simulink model "TestbedModel_v6"  (R2016a)
settings: Solver=ode23tb  StartTime=0.0  StopTime=20  RelTol=1e-3
undefined symbols (not defined in the file): K, Ki, Kp, magnitude, rev_comms_sink, tau
libraries: DAEMOT_Lib x4
(part 3 of 4)

== system TestbedModel_v6/Data Manager23 ==
  Bus Creator : BusCreator  Inputs=1
  Bus Selector1 : BusSelector  OutputSignals=Voltage [V]
  SubSystem1 : Subsystem
  Data : Outport
  wires:
  SubSystem1/1(Bus) -> Bus Creator/1  "Bus/Voltage [V]"
  Bus Selector1/1 -> SubSystem1/1(Rename)  "<Voltage [V]>"
  [gdata_BusData_Sink] -> Bus Selector1/1  "Bus/Voltage [V]"
  Bus Creator/1 -> Data/1

== system TestbedModel_v6/Data Manager24 ==
  Bus Creator : BusCreator  Inputs=1
  Bus Selector1 : BusSelector  OutputSignals=Speed [rad_s]
  SubSystem1 : Subsystem
  Data : Outport
  wires:
  Bus Creator/1 -> Data/1
  [gdata_ShaftData_Sink] -> Bus Selector1/1  "Shaft/Speed [rad_s]"
  Bus Selector1/1 -> SubSystem1/1(Rename)  "<Speed [rad_s]>"
  SubSystem1/1(Bus) -> Bus Creator/1  "Shaft/Speed [rad_s]"

== system TestbedModel_v6/Data Manager25 ==
  Bus Creator : BusCreator  Inputs=1
  Bus Selector1 : BusSelector  OutputSignals=Speed [rad_s]
  SubSystem1 : Subsystem
  Data : Outport
  wires:
  Bus Creator/1 -> Data/1
  [gdata_ShaftData_Sink] -> Bus Selector1/1  "Shaft/Speed [rad_s]"
  Bus Selector1/1 -> SubSystem1/1(Rename)  "<Speed [rad_s]>"
  SubSystem1/1(Bus) -> Bus Creator/1  "Shaft/Speed [rad_s]"

== system TestbedModel_v6/Data Manager3 ==
  Bus Creator : BusCreator  Inputs=1
  Bus Selector1 : BusSelector  OutputSignals=Voltage Out [V]
  SubSystem1 : Subsystem
  Data : Outport
  wires:
  Bus Creator/1 -> Data/1
  [gdata_ConverterData_Sink] -> Bus Selector1/1  "Converter/Voltage Out [V]"
  Bus Selector1/1 -> SubSystem1/1(Rename)  "<Voltage Out [V]>"
  SubSystem1/1(Bus) -> Bus Creator/1  "Converter/Voltage Out [V]"

== system TestbedModel_v6/Data Manager4 ==
  Bus Creator : BusCreator  Inputs=1
  Bus Selector1 : BusSelector  OutputSignals=Torque [Nm]
  SubSystem1 : Subsystem
  Data : Outport
  wires:
  Bus Creator/1 -> Data/1
  [gdata_MotorData_Sink] -> Bus Selector1/1  "Motor/Torque [Nm]"
  Bus Selector1/1 -> SubSystem1/1(Rename)  "<Torque [Nm]>"
  SubSystem1/1(Bus) -> Bus Creator/1  "Motor/Torque [Nm]"

== system TestbedModel_v6/Data Manager5 ==
  Bus Creator : BusCreator  Inputs=1
  Bus Selector1 : BusSelector  OutputSignals=Torque [Nm]
  SubSystem1 : Subsystem
  Data : Outport
  wires:
  Bus Creator/1 -> Data/1
  [gdata_MotorData_Sink] -> Bus Selector1/1  "Motor/Torque [Nm]"
  Bus Selector1/1 -> SubSystem1/1(Rename)  "<Torque [Nm]>"
  SubSystem1/1(Bus) -> Bus Creator/1  "Motor/Torque [Nm]"

== system TestbedModel_v6/Data Manager6 ==
  Bus Creator : BusCreator  Inputs=2
  Bus Selector1 : BusSelector  OutputSignals=Current In [A]
  Bus Selector2 : BusSelector  OutputSignals=Current In [A]
  SubSystem1 : Subsystem
  SubSystem2 : Subsystem
  Data : Outport
  wires:
  Bus Creator/1 -> Data/1
  [gdata_ConverterData_Sink] -> Bus Selector1/1  "Converter/Current In [A]"
  Bus Selector1/1 -> SubSystem1/1(Rename)  "<Current In [A]>"
  SubSystem1/1(Bus) -> Bus Creator/1  "Converter/Current In [A]"
  [gdata_Converter1Data_Sink] -> Bus Selector2/1  "Converter1/Current In [A]"
  Bus Selector2/1 -> SubSystem2/1(Rename)  "<Current In [A]>"
  SubSystem2/1(Bus) -> Bus Creator/2  "Converter1/Current In [A]"

== system TestbedModel_v6/Data Manager7 ==
  Bus Creator : BusCreator  Inputs=1
  Bus Selector1 : BusSelector  OutputSignals=Current1 [A]
  SubSystem1 : Subsystem
  Data : Outport
  wires:
  Bus Creator/1 -> Data/1
  [gdata_BusData_Sink] -> Bus Selector1/1  "Bus/Current1 [A]"
  Bus Selector1/1 -> SubSystem1/1(Rename)  "<Current1 [A]>"
  SubSystem1/1(Bus) -> Bus Creator/1  "Bus/Current1 [A]"

== system TestbedModel_v6/Data Manager8 ==
  Bus Creator : BusCreator  Inputs=1
  Bus Selector1 : BusSelector  OutputSignals=Voltage [V]
  SubSystem1 : Subsystem
  Data : Outport
  wires:
  Bus Creator/1 -> Data/1
  [gdata_BusData_Sink] -> Bus Selector1/1  "Bus/Voltage [V]"
  Bus Selector1/1 -> SubSystem1/1(Rename)  "<Voltage [V]>"
  SubSystem1/1(Bus) -> Bus Creator/1  "Bus/Voltage [V]"

== system TestbedModel_v6/Data Manager9 ==
  Bus Creator : BusCreator  Inputs=1
  Bus Selector1 : BusSelector  OutputSignals=Current [A]
  SubSystem1 : Subsystem
  Data : Outport
  wires:
  Bus Creator/1 -> Data/1
  [gdata_Motor1Data_Sink] -> Bus Selector1/1  "Motor1/Current [A]"
  Bus Selector1/1 -> SubSystem1/1(Rename)  "<Current [A]>"
  SubSystem1/1(Bus) -> Bus Creator/1  "Motor1/Current [A]"

== system TestbedModel_v6/Effort Sink1 ==
  In1 : Inport
  Sink1 : Subsystem  LoadFcn=rev_comms_sink();  InitFcn=rev_comms_sink();  mask(Sink){}
      mask help: Used for sending data to the upstream component.
      settings: CopyFcn=rev_comms_sink();  NameChangeFcn=rev_comms_sink();
      mask Display: text(0.25,0.5,'Sink')
  Terminator : Terminator
  val : Constant  Value=value
  wires:
  val/1 -> Sink1/1(In1)
  In1/1 -> Terminator/1

== system TestbedModel_v6/Effort Sink10 ==
  In1 : Inport
  In2 : Inport  Port=2
  Sink1 : Subsystem  LoadFcn=rev_comms_sink();  InitFcn=rev_comms_sink();  mask(Sink){}
      mask help: Used for sending data to the upstream component.
      settings: CopyFcn=rev_comms_sink();  NameChangeFcn=rev_comms_sink();
      mask Display: text(0.25,0.5,'Sink')
  Terminator : Terminator
  wires:
  In1/1 -> Terminator/1
  In2/1 -> Sink1/1(In1)

== system TestbedModel_v6/Effort Sink11 ==
  In1 : Inport
  Sink1 : Subsystem  LoadFcn=rev_comms_sink();  InitFcn=rev_comms_sink();  mask(Sink){}
      mask help: Used for sending data to the upstream component.
      settings: CopyFcn=rev_comms_sink();  NameChangeFcn=rev_comms_sink();
      mask Display: text(0.25,0.5,'Sink')
  Terminator : Terminator
  val : Constant  Value=value
  wires:
  val/1 -> Sink1/1(In1)
  In1/1 -> Terminator/1

== system TestbedModel_v6/Effort Sink12 ==
  In1 : Inport
  Sink1 : Subsystem  LoadFcn=rev_comms_sink();  InitFcn=rev_comms_sink();  mask(Sink){}
      mask help: Used for sending data to the upstream component.
      settings: CopyFcn=rev_comms_sink();  NameChangeFcn=rev_comms_sink();
      mask Display: text(0.25,0.5,'Sink')
  Terminator : Terminator
  val : Constant  Value=value
  wires:
  val/1 -> Sink1/1(In1)
  In1/1 -> Terminator/1

== system TestbedModel_v6/Effort Sink13 ==
  In1 : Inport
  In2 : Inport  Port=2
  Sink1 : Subsystem  LoadFcn=rev_comms_sink();  InitFcn=rev_comms_sink();  mask(Sink){}
      mask help: Used for sending data to the upstream component.
      settings: CopyFcn=rev_comms_sink();  NameChangeFcn=rev_comms_sink();
      mask Display: text(0.25,0.5,'Sink')
  Terminator : Terminator
  wires:
  In1/1 -> Terminator/1
  In2/1 -> Sink1/1(In1)

== system TestbedModel_v6/Effort Sink14 ==
  In1 : Inport
  Sink1 : Subsystem  LoadFcn=rev_comms_sink();  InitFcn=rev_comms_sink();  mask(Sink){}
      mask help: Used for sending data to the upstream component.
      settings: CopyFcn=rev_comms_sink();  NameChangeFcn=rev_comms_sink();
      mask Display: text(0.25,0.5,'Sink')
  Terminator : Terminator
  val : Constant  Value=value
  wires:
  In1/1 -> Terminator/1
  val/1 -> Sink1/1(In1)

== system TestbedModel_v6/Effort Sink15 ==
  In1 : Inport
  Sink1 : Subsystem  LoadFcn=rev_comms_sink();  InitFcn=rev_comms_sink();  mask(Sink){}
      mask help: Used for sending data to the upstream component.
      settings: CopyFcn=rev_comms_sink();  NameChangeFcn=rev_comms_sink();
      mask Display: text(0.25,0.5,'Sink')
  Terminator : Terminator
  val : Constant  Value=value
  wires:
  In1/1 -> Terminator/1
  val/1 -> Sink1/1(In1)

== system TestbedModel_v6/Effort Sink16 ==
  In1 : Inport
  In2 : Inport  Port=2
  Sink1 : Subsystem  LoadFcn=rev_comms_sink();  InitFcn=rev_comms_sink();  mask(Sink){}
      mask help: Used for sending data to the upstream component.
      settings: CopyFcn=rev_comms_sink();  NameChangeFcn=rev_comms_sink();
      mask Display: text(0.25,0.5,'Sink')
  Terminator : Terminator
  wires:
  In2/1 -> Sink1/1(In1)
  In1/1 -> Terminator/1

== system TestbedModel_v6/Effort Sink2 ==
  In1 : Inport
  Sink1 : Subsystem  LoadFcn=rev_comms_sink();  InitFcn=rev_comms_sink();  mask(Sink){}
      mask help: Used for sending data to the upstream component.
      settings: CopyFcn=rev_comms_sink();  NameChangeFcn=rev_comms_sink();
      mask Display: text(0.25,0.5,'Sink')
  Terminator : Terminator
  val : Constant  Value=value
  wires:
  In1/1 -> Terminator/1
  val/1 -> Sink1/1(In1)

== system TestbedModel_v6/Effort Sink3 ==
  In1 : Inport
  Sink1 : Subsystem  LoadFcn=rev_comms_sink();  InitFcn=rev_comms_sink();  mask(Sink){}
      mask help: Used for sending data to the upstream component.
      settings: CopyFcn=rev_comms_sink();  NameChangeFcn=rev_comms_sink();
      mask Display: text(0.25,0.5,'Sink')
  Terminator : Terminator
  val : Constant  Value=value
  wires:
  val/1 -> Sink1/1(In1)
  In1/1 -> Terminator/1

== system TestbedModel_v6/Effort Sink4 ==
  In1 : Inport
  Sink1 : Subsystem  LoadFcn=rev_comms_sink();  InitFcn=rev_comms_sink();  mask(Sink){}
      mask help: Used for sending data to the upstream component.
      settings: CopyFcn=rev_comms_sink();  NameChangeFcn=rev_comms_sink();
      mask Display: text(0.25,0.5,'Sink')
  Terminator : Terminator
  val : Constant  Value=value
  wires:
  val/1 -> Sink1/1(In1)
  In1/1 -> Terminator/1

== system TestbedModel_v6/Effort Sink5 ==
  In1 : Inport
  Sink1 : Subsystem  LoadFcn=rev_comms_sink();  InitFcn=rev_comms_sink();  mask(Sink){}
      mask help: Used for sending data to the upstream component.
      settings: CopyFcn=rev_comms_sink();  NameChangeFcn=rev_comms_sink();
      mask Display: text(0.25,0.5,'Sink')
  Terminator : Terminator
  val : Constant  Value=value
  wires:
  In1/1 -> Terminator/1
  val/1 -> Sink1/1(In1)

== system TestbedModel_v6/Effort Sink6 ==
  In1 : Inport
  In2 : Inport  Port=2
  Sink1 : Subsystem  LoadFcn=rev_comms_sink();  InitFcn=rev_comms_sink();  mask(Sink){}
      mask help: Used for sending data to the upstream component.
      settings: CopyFcn=rev_comms_sink();  NameChangeFcn=rev_comms_sink();
      mask Display: text(0.25,0.5,'Sink')
  Terminator : Terminator
  wires:
  In1/1 -> Terminator/1
  In2/1 -> Sink1/1(In1)

== system TestbedModel_v6/Effort Sink7 ==
  In1 : Inport
  Sink1 : Subsystem  LoadFcn=rev_comms_sink();  InitFcn=rev_comms_sink();  mask(Sink){}
      mask help: Used for sending data to the upstream component.
      settings: CopyFcn=rev_comms_sink();  NameChangeFcn=rev_comms_sink();
      mask Display: text(0.25,0.5,'Sink')
  Terminator : Terminator
  val : Constant  Value=value
  wires:
  In1/1 -> Terminator/1
  val/1 -> Sink1/1(In1)

== system TestbedModel_v6/Effort Sink8 ==
  In1 : Inport
  Sink1 : Subsystem  LoadFcn=rev_comms_sink();  InitFcn=rev_comms_sink();  mask(Sink){}
      mask help: Used for sending data to the upstream component.
      settings: CopyFcn=rev_comms_sink();  NameChangeFcn=rev_comms_sink();
      mask Display: text(0.25,0.5,'Sink')
  Terminator : Terminator
  val : Constant  Value=value
  wires:
  val/1 -> Sink1/1(In1)
  In1/1 -> Terminator/1

== system TestbedModel_v6/Effort Sink9 ==
  In1 : Inport
  In2 : Inport  Port=2
  Sink1 : Subsystem  LoadFcn=rev_comms_sink();  InitFcn=rev_comms_sink();  mask(Sink){}
      mask help: Used for sending data to the upstream component.
      settings: CopyFcn=rev_comms_sink();  NameChangeFcn=rev_comms_sink();
      mask Display: text(0.25,0.5,'Sink')
  Terminator : Terminator
  wires:
  In1/1 -> Terminator/1
  In2/1 -> Sink1/1(In1)

== system TestbedModel_v6/Effort Source ==
  Constant : Constant  Value=0
  Source1 : Subsystem  mask(Source){}
      mask help: Used for receiving data from the downstream component.
      mask init:
      | n_src = gcb;
      | n_src = str2num(n_src(end));
      | try
      |     rev_comms_source(n_src);
      | catch
      | 
      | end
      mask Display: text(0.25,0.5,'Source')
  Terminator : Terminator
  b1 : BusCreator  Inputs=2
  val : Constant  Value=value
  Out1 : Outport
  wires:
  b1/1 -> Out1/1
  Source1/1(Out1) -> Terminator/1
  Constant/1 -> b1/1  "current"
  val/1 -> b1/2  "voltage"

== system TestbedModel_v6/Effort Source1 ==
  In1 : Inport
  Constant : Constant  Value=0
  Source1 : Subsystem  mask(Source){}
      mask help: Used for receiving data from the downstream component.
      mask init:
      | n_src = gcb;
      | n_src = str2num(n_src(end));
      | try
      |     rev_comms_source(n_src);
      | catch
      | 
      | end
      mask Display: text(0.25,0.5,'Source')
  Terminator : Terminator
  b1 : BusCreator  Inputs=2
  Out1 : Outport
  wires:
  Constant/1 -> b1/1  "current"
  Source1/1(Out1) -> Terminator/1
  b1/1 -> Out1/1
  In1/1 -> b1/2  "voltage"

== system TestbedModel_v6/Inductor ==
  In1 : Inport
  Bus Creator1 : BusCreator  Inputs=1
  Bus Creator3 : BusCreator  Inputs=2
  Bus Selector1 : BusSelector  OutputSignals=current,voltage
  Current : MATLAB Function  TreatAsAtomicUnit=on
  Data_Sink : Subsystem  LoadFcn=|  InitFcn=|  mask(Data Sink){}
      LoadFcn=|
      | h      = get_param(gcb,'handle');   % Get block handle                           
      | hblock = get(h);     % Parse out handles structure
      | 
      | str = [hblock.Path(numel(bdroot)+2:end), hblock.Name];
      | str(~ismember(str,['A':'Z' 'a':'z' '0':'9' '_'])) = '';                     
      | set_param([gcb, '/global_data_goto'],'GotoTag',['gdata_',str]);
      |                                
      |                                                                                  
      | clear h hblock str
      InitFcn=|
      | h      = get_param(gcb,'handle');   % Get block handle                           
      | hblock = get(h);     % Parse out handles structure
      | 
      | str = [hblock.Path(numel(bdroot)+2:end), hblock.Name];
      | str(~ismember(str,['A':'Z' 'a':'z' '0':'9' '_'])) = '';                     
      | set_param([gcb, '/global_data_goto'],'GotoTag',['gdata_',str]);
      |                                
      |                                                                                  
      | clear h hblock str
      mask help:
      | Input to this block should be a bus signal with named signals.
      |
      | Bus signals sent to this block will be read by the Data Manager.
      | The Data Manager will handle the global routing of signals.
      |
      | This block should be placed under the mask of components.
      settings: CopyFcn=|
      | h      = get_param(gcb,'handle');   % Get block handle
      | hblock = get(h);     % Parse out handles structure
      | 
      | str = [hblock.Path(numel(bdroot)+2:end), hblock.Name];
      | str(~ismember(str,['A':'Z' 'a':'z' '0':'9' '_'])) = '';
      | set_param([gcb, '/global_data_goto'],'GotoTag',['gdata_',str]);
      | 
      | 
      | clear h hblock str
      settings: NameChangeFcn=|
      | h      = get_param(gcb,'handle');   % Get block handle
      | hblock = get(h);     % Parse out handles structure
      | 
      | str = [hblock.Path(numel(bdroot)+2:end), hblock.Name];
      | str(~ismember(str,['A':'Z' 'a':'z' '0':'9' '_'])) = '';
      | set_param([gcb, '/global_data_goto'],'GotoTag',['gdata_',str]);
      | 
      | 
      | clear h hblock str
      mask Display: text(0.25,0.5,'Data Sink')
  Integrator3 : Integrator  InitialCondition=I_initial
  Sink1 : Subsystem  LoadFcn=rev_comms_sink();  InitFcn=rev_comms_sink();  mask(Sink){}
      mask help: Used for sending data to the upstream component.
      settings: CopyFcn=rev_comms_sink();  NameChangeFcn=rev_comms_sink();
      mask Display: text(0.25,0.5,'Sink')
  Source1 : Subsystem  mask(Source){}
      mask help: Used for receiving data from the downstream component.
      mask init:
      | n_src = gcb;
      | n_src = str2num(n_src(end));
      | try
      |     rev_comms_source(n_src);
      | catch
      | 
      | end
      mask Display: text(0.25,0.5,'Source')
  Terminator : Terminator
  Out1 : Outport
  wires:
  [I] -> Bus Creator1/1  "Current [A]"
  Bus Creator1/1 -> Data_Sink/1(" ")
  Integrator3/1 -> [I]
  Current/1(dI_dt) -> Integrator3/1
  [V_out] -> Current/2(V_out)
  [V_in] -> Current/1(V_in)
  [I] -> Bus Creator3/1  "current"
  Source1/1(Out1) -> [V_out]
  Bus Selector1/1 -> Terminator/1  "<current>"
  Bus Selector1/2 -> [V_in]  "<voltage>"
  [V_out] -> Bus Creator3/2  "voltage"
  [I] -> Sink1/1(In1)
  In1/1 -> Bus Selector1/1  "electric"
  Bus Creator3/1 -> Out1/1

== system TestbedModel_v6/Inductor1 ==
  In1 : Inport
  Bus Creator1 : BusCreator  Inputs=1
  Bus Creator3 : BusCreator  Inputs=2
  Bus Selector1 : BusSelector  OutputSignals=current,voltage
  Current : MATLAB Function  TreatAsAtomicUnit=on
  Data_Sink : Subsystem  LoadFcn=|  InitFcn=|  mask(Data Sink){}
      LoadFcn=|
      | h      = get_param(gcb,'handle');   % Get block handle                           
      | hblock = get(h);     % Parse out handles structure
      | 
      | str = [hblock.Path(numel(bdroot)+2:end), hblock.Name];
      | str(~ismember(str,['A':'Z' 'a':'z' '0':'9' '_'])) = '';                     
      | set_param([gcb, '/global_data_goto'],'GotoTag',['gdata_',str]);
      |                                
      |                                                                                  
      | clear h hblock str
      InitFcn=|
      | h      = get_param(gcb,'handle');   % Get block handle                           
      | hblock = get(h);     % Parse out handles structure
      | 
      | str = [hblock.Path(numel(bdroot)+2:end), hblock.Name];
      | str(~ismember(str,['A':'Z' 'a':'z' '0':'9' '_'])) = '';                     
      | set_param([gcb, '/global_data_goto'],'GotoTag',['gdata_',str]);
      |                                
      |                                                                                  
      | clear h hblock str
      mask help:
      | Input to this block should be a bus signal with named signals.
      |
      | Bus signals sent to this block will be read by the Data Manager.
      | The Data Manager will handle the global routing of signals.
      |
      | This block should be placed under the mask of components.
      settings: CopyFcn=|
      | h      = get_param(gcb,'handle');   % Get block handle
      | hblock = get(h);     % Parse out handles structure
      | 
      | str = [hblock.Path(numel(bdroot)+2:end), hblock.Name];
      | str(~ismember(str,['A':'Z' 'a':'z' '0':'9' '_'])) = '';
      | set_param([gcb, '/global_data_goto'],'GotoTag',['gdata_',str]);
      | 
      | 
      | clear h hblock str
      settings: NameChangeFcn=|
      | h      = get_param(gcb,'handle');   % Get block handle
      | hblock = get(h);     % Parse out handles structure
      | 
      | str = [hblock.Path(numel(bdroot)+2:end), hblock.Name];
      | str(~ismember(str,['A':'Z' 'a':'z' '0':'9' '_'])) = '';
      | set_param([gcb, '/global_data_goto'],'GotoTag',['gdata_',str]);
      | 
      | 
      | clear h hblock str
      mask Display: text(0.25,0.5,'Data Sink')
  Integrator3 : Integrator  InitialCondition=I_initial
  Sink1 : Subsystem  LoadFcn=rev_comms_sink();  InitFcn=rev_comms_sink();  mask(Sink){}
      mask help: Used for sending data to the upstream component.
      settings: CopyFcn=rev_comms_sink();  NameChangeFcn=rev_comms_sink();
      mask Display: text(0.25,0.5,'Sink')
  Source1 : Subsystem  mask(Source){}
      mask help: Used for receiving data from the downstream component.
      mask init:
      | n_src = gcb;
      | n_src = str2num(n_src(end));
      | try
      |     rev_comms_source(n_src);
      | catch
      | 
      | end
      mask Display: text(0.25,0.5,'Source')
  Terminator : Terminator
  Out1 : Outport
  wires:
  Bus Creator3/1 -> Out1/1
  In1/1 -> Bus Selector1/1  "electric"
  [I] -> Sink1/1(In1)
  [V_out] -> Bus Creator3/2  "voltage"
  Bus Selector1/2 -> [V_in]  "<voltage>"
  Bus Selector1/1 -> Terminator/1  "<current>"
  Source1/1(Out1) -> [V_out]
  [I] -> Bus Creator3/1  "current"
  [V_in] -> Current/1(V_in)
  [V_out] -> Current/2(V_out)
  Current/1(dI_dt) -> Integrator3/1
  Integrator3/1 -> [I]
  Bus Creator1/1 -> Data_Sink/1(" ")
  [I] -> Bus Creator1/1  "Current [A]"

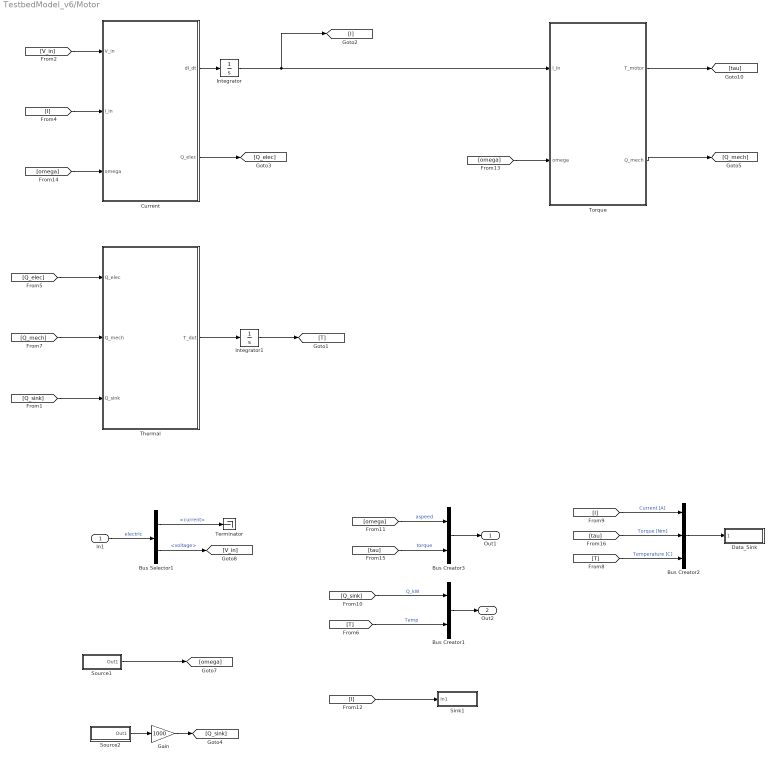
== system TestbedModel_v6/Motor ==
  In1 : Inport
  Bus Creator1 : BusCreator  Inputs=2
  Bus Creator2 : BusCreator  Inputs=3
  Bus Creator3 : BusCreator  Inputs=2
  Bus Selector1 : BusSelector  OutputSignals=current,voltage
  Current : MATLAB Function  TreatAsAtomicUnit=on
  Data_Sink : Subsystem  LoadFcn=|  InitFcn=|  mask(Data Sink){}
      LoadFcn=|
      | h      = get_param(gcb,'handle');   % Get block handle                           
      | hblock = get(h);     % Parse out handles structure
      | 
      | str = [hblock.Path(numel(bdroot)+2:end), hblock.Name];
      | str(~ismember(str,['A':'Z' 'a':'z' '0':'9' '_'])) = '';                     
      | set_param([gcb, '/global_data_goto'],'GotoTag',['gdata_',str]);
      |                                
      |                                                                                  
      | clear h hblock str
      InitFcn=|
      | h      = get_param(gcb,'handle');   % Get block handle                           
      | hblock = get(h);     % Parse out handles structure
      | 
      | str = [hblock.Path(numel(bdroot)+2:end), hblock.Name];
      | str(~ismember(str,['A':'Z' 'a':'z' '0':'9' '_'])) = '';                     
      | set_param([gcb, '/global_data_goto'],'GotoTag',['gdata_',str]);
      |                                
      |                                                                                  
      | clear h hblock str
      mask help:
      | Input to this block should be a bus signal with named signals.
      |
      | Bus signals sent to this block will be read by the Data Manager.
      | The Data Manager will handle the global routing of signals.
      |
      | This block should be placed under the mask of components.
      settings: CopyFcn=|
      | h      = get_param(gcb,'handle');   % Get block handle
      | hblock = get(h);     % Parse out handles structure
      | 
      | str = [hblock.Path(numel(bdroot)+2:end), hblock.Name];
      | str(~ismember(str,['A':'Z' 'a':'z' '0':'9' '_'])) = '';
      | set_param([gcb, '/global_data_goto'],'GotoTag',['gdata_',str]);
      | 
      | 
      | clear h hblock str
      settings: NameChangeFcn=|
      | h      = get_param(gcb,'handle');   % Get block handle
      | hblock = get(h);     % Parse out handles structure
      | 
      | str = [hblock.Path(numel(bdroot)+2:end), hblock.Name];
      | str(~ismember(str,['A':'Z' 'a':'z' '0':'9' '_'])) = '';
      | set_param([gcb, '/global_data_goto'],'GotoTag',['gdata_',str]);
      | 
      | 
      | clear h hblock str
      mask Display: text(0.25,0.5,'Data Sink')
  Gain : Gain  Gain=1000
  Integrator : Integrator  InitialCondition=I_initial
  Integrator1 : Integrator  InitialCondition=T_initial
  Sink1 : Subsystem  LoadFcn=rev_comms_sink();  InitFcn=rev_comms_sink();  mask(Sink){}
      mask help: Used for sending data to the upstream component.
      settings: CopyFcn=rev_comms_sink();  NameChangeFcn=rev_comms_sink();
      mask Display: text(0.25,0.5,'Sink')
  Source1 : Subsystem  mask(Source){}
      mask help: Used for receiving data from the downstream component.
      mask init:
      | n_src = gcb;
      | n_src = str2num(n_src(end));
      | try
      |     rev_comms_source(n_src);
      | catch
      | 
      | end
      mask Display: text(0.25,0.5,'Source')
  Source2 : Subsystem  mask(Source){}
      mask help: Used for receiving data from the downstream component.
      mask init:
      | n_src = gcb;
      | n_src = str2num(n_src(end));
      | try
      |     rev_comms_source(n_src);
      | catch
      | 
      | end
      mask Display: text(0.25,0.5,'Source')
  Terminator : Terminator
  Thermal : MATLAB Function  TreatAsAtomicUnit=on
  Torque : MATLAB Function  TreatAsAtomicUnit=on
  Out1 : Outport
  Out2 : Outport  Port=2
  wires:
  Gain/1 -> [Q_sink]
  [Q_sink] -> Bus Creator1/1  "Q_kW"
  [T] -> Bus Creator1/2  "Temp"
  Bus Creator1/1 -> Out2/1
  [Q_mech] -> Thermal/2(Q_mech)
  Torque/2(Q_mech) -> [Q_mech]
  [omega] -> Torque/2(omega)
  Source1/1(Out1) -> [omega]
  Source2/1(Out1) -> Gain/1
  [V_in] -> Current/1(V_in)
  Integrator/1 -> [I], Torque/1(I_in)
  [T] -> Bus Creator2/3  "Temperature [C]"
  [tau] -> Bus Creator2/2  "Torque [Nm]"
  Bus Creator2/1 -> Data_Sink/1(" ")
  [omega] -> Current/3(omega)
  Bus Selector1/1 -> Terminator/1  "<current>"
  Bus Selector1/2 -> [V_in]  "<voltage>"
  [omega] -> Bus Creator3/1  "aspeed"
  [I] -> Sink1/1(In1)
  In1/1 -> Bus Selector1/1  "electric"
  Bus Creator3/1 -> Out1/1
  Current/1(dI_dt) -> Integrator/1
  [I] -> Current/2(I_in)
  Thermal/1(T_dot) -> Integrator1/1
  Integrator1/1 -> [T]
  Current/2(Q_elec) -> [Q_elec]
  [Q_elec] -> Thermal/1(Q_elec)
  [Q_sink] -> Thermal/3(Q_sink)
  Torque/1(T_motor) -> [tau]
  [tau] -> Bus Creator3/2  "torque"
  [I] -> Bus Creator2/1  "Current [A]"

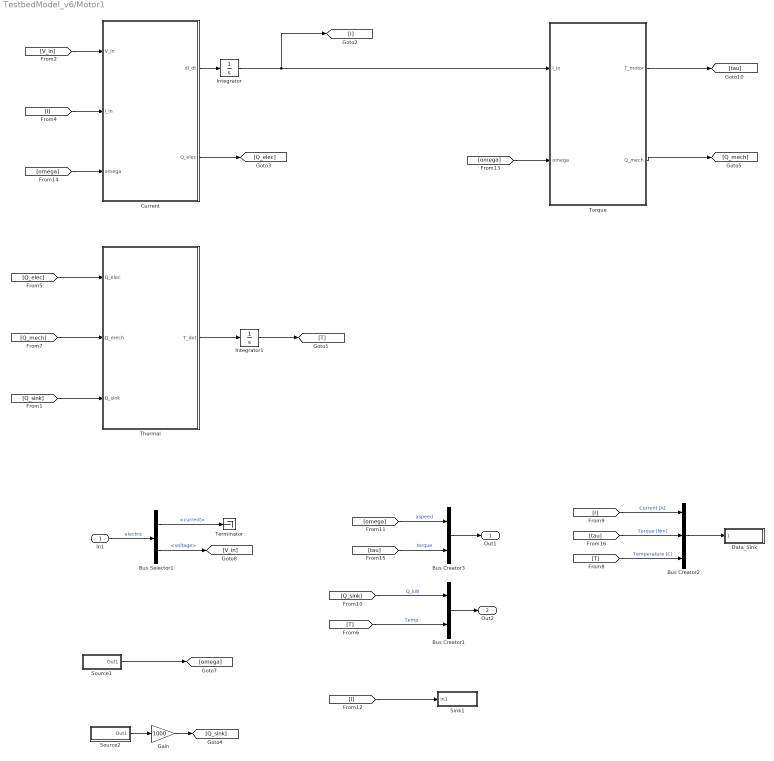
== system TestbedModel_v6/Motor1 ==
  In1 : Inport
  Bus Creator1 : BusCreator  Inputs=2
  Bus Creator2 : BusCreator  Inputs=3
  Bus Creator3 : BusCreator  Inputs=2
  Bus Selector1 : BusSelector  OutputSignals=current,voltage
  Current : MATLAB Function  TreatAsAtomicUnit=on
  Data_Sink : Subsystem  LoadFcn=|  InitFcn=|  mask(Data Sink){}
      LoadFcn=|
      | h      = get_param(gcb,'handle');   % Get block handle                           
      | hblock = get(h);     % Parse out handles structure
      | 
      | str = [hblock.Path(numel(bdroot)+2:end), hblock.Name];
      | str(~ismember(str,['A':'Z' 'a':'z' '0':'9' '_'])) = '';                     
      | set_param([gcb, '/global_data_goto'],'GotoTag',['gdata_',str]);
      |                                
      |                                                                                  
      | clear h hblock str
      InitFcn=|
      | h      = get_param(gcb,'handle');   % Get block handle                           
      | hblock = get(h);     % Parse out handles structure
      | 
      | str = [hblock.Path(numel(bdroot)+2:end), hblock.Name];
      | str(~ismember(str,['A':'Z' 'a':'z' '0':'9' '_'])) = '';                     
      | set_param([gcb, '/global_data_goto'],'GotoTag',['gdata_',str]);
      |                                
      |                                                                                  
      | clear h hblock str
      mask help:
      | Input to this block should be a bus signal with named signals.
      |
      | Bus signals sent to this block will be read by the Data Manager.
      | The Data Manager will handle the global routing of signals.
      |
      | This block should be placed under the mask of components.
      settings: CopyFcn=|
      | h      = get_param(gcb,'handle');   % Get block handle
      | hblock = get(h);     % Parse out handles structure
      | 
      | str = [hblock.Path(numel(bdroot)+2:end), hblock.Name];
      | str(~ismember(str,['A':'Z' 'a':'z' '0':'9' '_'])) = '';
      | set_param([gcb, '/global_data_goto'],'GotoTag',['gdata_',str]);
      | 
      | 
      | clear h hblock str
      settings: NameChangeFcn=|
      | h      = get_param(gcb,'handle');   % Get block handle
      | hblock = get(h);     % Parse out handles structure
      | 
      | str = [hblock.Path(numel(bdroot)+2:end), hblock.Name];
      | str(~ismember(str,['A':'Z' 'a':'z' '0':'9' '_'])) = '';
      | set_param([gcb, '/global_data_goto'],'GotoTag',['gdata_',str]);
      | 
      | 
      | clear h hblock str
      mask Display: text(0.25,0.5,'Data Sink')
  Gain : Gain  Gain=1000
  Integrator : Integrator  InitialCondition=I_initial
  Integrator1 : Integrator  InitialCondition=T_initial
  Sink1 : Subsystem  LoadFcn=rev_comms_sink();  InitFcn=rev_comms_sink();  mask(Sink){}
      mask help: Used for sending data to the upstream component.
      settings: CopyFcn=rev_comms_sink();  NameChangeFcn=rev_comms_sink();
      mask Display: text(0.25,0.5,'Sink')
  Source1 : Subsystem  mask(Source){}
      mask help: Used for receiving data from the downstream component.
      mask init:
      | n_src = gcb;
      | n_src = str2num(n_src(end));
      | try
      |     rev_comms_source(n_src);
      | catch
      | 
      | end
      mask Display: text(0.25,0.5,'Source')
  Source2 : Subsystem  mask(Source){}
      mask help: Used for receiving data from the downstream component.
      mask init:
      | n_src = gcb;
      | n_src = str2num(n_src(end));
      | try
      |     rev_comms_source(n_src);
      | catch
      | 
      | end
      mask Display: text(0.25,0.5,'Source')
  Terminator : Terminator
  Thermal : MATLAB Function  TreatAsAtomicUnit=on
  Torque : MATLAB Function  TreatAsAtomicUnit=on
  Out1 : Outport
  Out2 : Outport  Port=2
  wires:
  Gain/1 -> [Q_sink]
  [Q_sink] -> Bus Creator1/1  "Q_kW"
  [T] -> Bus Creator1/2  "Temp"
  Bus Creator1/1 -> Out2/1
  [Q_mech] -> Thermal/2(Q_mech)
  Torque/2(Q_mech) -> [Q_mech]
  [omega] -> Torque/2(omega)
  Source1/1(Out1) -> [omega]
  Source2/1(Out1) -> Gain/1
  [V_in] -> Current/1(V_in)
  Integrator/1 -> [I], Torque/1(I_in)
  [T] -> Bus Creator2/3  "Temperature [C]"
  [tau] -> Bus Creator2/2  "Torque [Nm]"
  Bus Creator2/1 -> Data_Sink/1(" ")
  [omega] -> Current/3(omega)
  Bus Selector1/1 -> Terminator/1  "<current>"
  Bus Selector1/2 -> [V_in]  "<voltage>"
  [omega] -> Bus Creator3/1  "aspeed"
  [I] -> Sink1/1(In1)
  In1/1 -> Bus Selector1/1  "electric"
  Bus Creator3/1 -> Out1/1
  Current/1(dI_dt) -> Integrator/1
  [I] -> Current/2(I_in)
  Thermal/1(T_dot) -> Integrator1/1
  Integrator1/1 -> [T]
  Current/2(Q_elec) -> [Q_elec]
  [Q_elec] -> Thermal/1(Q_elec)
  [Q_sink] -> Thermal/3(Q_sink)
  Torque/1(T_motor) -> [tau]
  [tau] -> Bus Creator3/2  "torque"
  [I] -> Bus Creator2/1  "Current [A]"

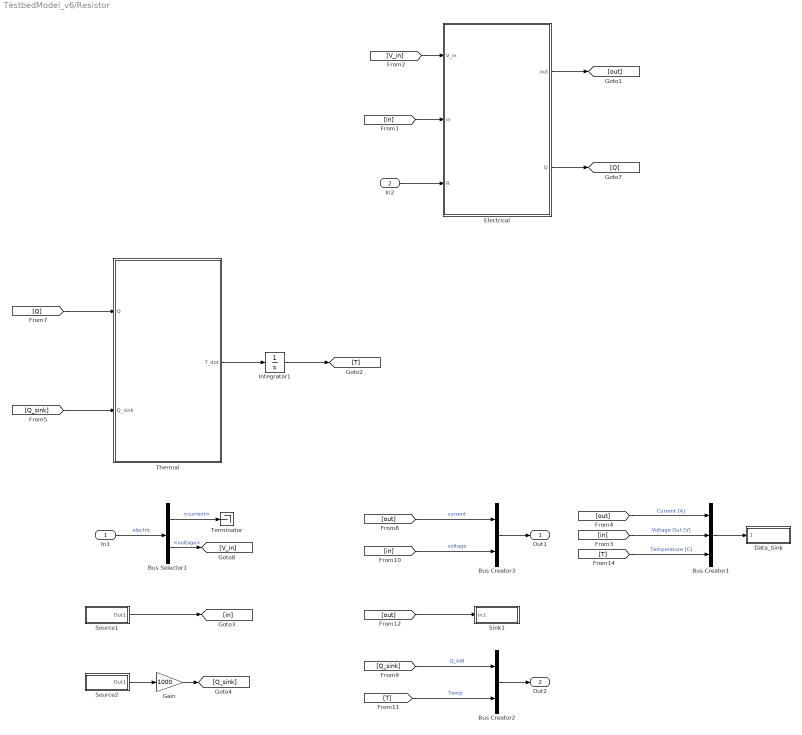
== system TestbedModel_v6/Resistor ==
  In1 : Inport
  In2 : Inport  Port=2
  Bus Creator1 : BusCreator  Inputs=3
  Bus Creator2 : BusCreator  Inputs=2
  Bus Creator3 : BusCreator  Inputs=2
  Bus Selector1 : BusSelector  OutputSignals=current,voltage
  Data_Sink : Subsystem  LoadFcn=|  InitFcn=|  mask(Data Sink){}
      LoadFcn=|
      | h      = get_param(gcb,'handle');   % Get block handle                           
      | hblock = get(h);     % Parse out handles structure
      | 
      | str = [hblock.Path(numel(bdroot)+2:end), hblock.Name];
      | str(~ismember(str,['A':'Z' 'a':'z' '0':'9' '_'])) = '';                     
      | set_param([gcb, '/global_data_goto'],'GotoTag',['gdata_',str]);
      |                                
      |                                                                                  
      | clear h hblock str
      InitFcn=|
      | h      = get_param(gcb,'handle');   % Get block handle                           
      | hblock = get(h);     % Parse out handles structure
      | 
      | str = [hblock.Path(numel(bdroot)+2:end), hblock.Name];
      | str(~ismember(str,['A':'Z' 'a':'z' '0':'9' '_'])) = '';                     
      | set_param([gcb, '/global_data_goto'],'GotoTag',['gdata_',str]);
      |                                
      |                                                                                  
      | clear h hblock str
      mask help:
      | Input to this block should be a bus signal with named signals.
      |
      | Bus signals sent to this block will be read by the Data Manager.
      | The Data Manager will handle the global routing of signals.
      |
      | This block should be placed under the mask of components.
      settings: CopyFcn=|
      | h      = get_param(gcb,'handle');   % Get block handle
      | hblock = get(h);     % Parse out handles structure
      | 
      | str = [hblock.Path(numel(bdroot)+2:end), hblock.Name];
      | str(~ismember(str,['A':'Z' 'a':'z' '0':'9' '_'])) = '';
      | set_param([gcb, '/global_data_goto'],'GotoTag',['gdata_',str]);
      | 
      | 
      | clear h hblock str
      settings: NameChangeFcn=|
      | h      = get_param(gcb,'handle');   % Get block handle
      | hblock = get(h);     % Parse out handles structure
      | 
      | str = [hblock.Path(numel(bdroot)+2:end), hblock.Name];
      | str(~ismember(str,['A':'Z' 'a':'z' '0':'9' '_'])) = '';
      | set_param([gcb, '/global_data_goto'],'GotoTag',['gdata_',str]);
      | 
      | 
      | clear h hblock str
      mask Display: text(0.25,0.5,'Data Sink')
  Electrical : MATLAB Function  TreatAsAtomicUnit=on
  Gain : Gain  Gain=1000
  Integrator1 : Integrator  InitialCondition=T_initial
  Sink1 : Subsystem  LoadFcn=rev_comms_sink();  InitFcn=rev_comms_sink();  mask(Sink){}
      mask help: Used for sending data to the upstream component.
      settings: CopyFcn=rev_comms_sink();  NameChangeFcn=rev_comms_sink();
      mask Display: text(0.25,0.5,'Sink')
  Source1 : Subsystem  mask(Source){}
      mask help: Used for receiving data from the downstream component.
      mask init:
      | n_src = gcb;
      | n_src = str2num(n_src(end));
      | try
      |     rev_comms_source(n_src);
      | catch
      | 
      | end
      mask Display: text(0.25,0.5,'Source')
  Source2 : Subsystem  mask(Source){}
      mask help: Used for receiving data from the downstream component.
      mask init:
      | n_src = gcb;
      | n_src = str2num(n_src(end));
      | try
      |     rev_comms_source(n_src);
      | catch
      | 
      | end
      mask Display: text(0.25,0.5,'Source')
  Terminator : Terminator
  Thermal : MATLAB Function  TreatAsAtomicUnit=on
  Out1 : Outport
  Out2 : Outport  Port=2
  wires:
  Gain/1 -> [Q_sink]
  [Q_sink] -> Bus Creator2/1  "Q_kW"
  [T] -> Bus Creator2/2  "Temp"
  Bus Creator2/1 -> Out2/1
  [out] -> Bus Creator3/1  "current"
  Source1/1(Out1) -> [in]
  Bus Selector1/1 -> Terminator/1  "<current>"
  Bus Selector1/2 -> [V_in]  "<voltage>"
  [in] -> Bus Creator3/2  "voltage"
  [out] -> Sink1/1(In1)
  In1/1 -> Bus Selector1/1  "electric"
  Electrical/1(out) -> [out]
  Bus Creator3/1 -> Out1/1
  [V_in] -> Electrical/1(V_in)
  [in] -> Electrical/2(in)
  [out] -> Bus Creator1/1  "Current [A]"
  [in] -> Bus Creator1/2  "Voltage Out [V]"
  Bus Creator1/1 -> Data_Sink/1(" ")
  [Q_sink] -> Thermal/2(Q_sink)
  [Q] -> Thermal/1(Q)
  Integrator1/1 -> [T]
  Thermal/1(T_dot) -> Integrator1/1
  Electrical/2(Q) -> [Q]
  [T] -> Bus Creator1/3  "Temperature [C]"
  Source2/1(Out1) -> Gain/1
  In2/1 -> Electrical/3(R)

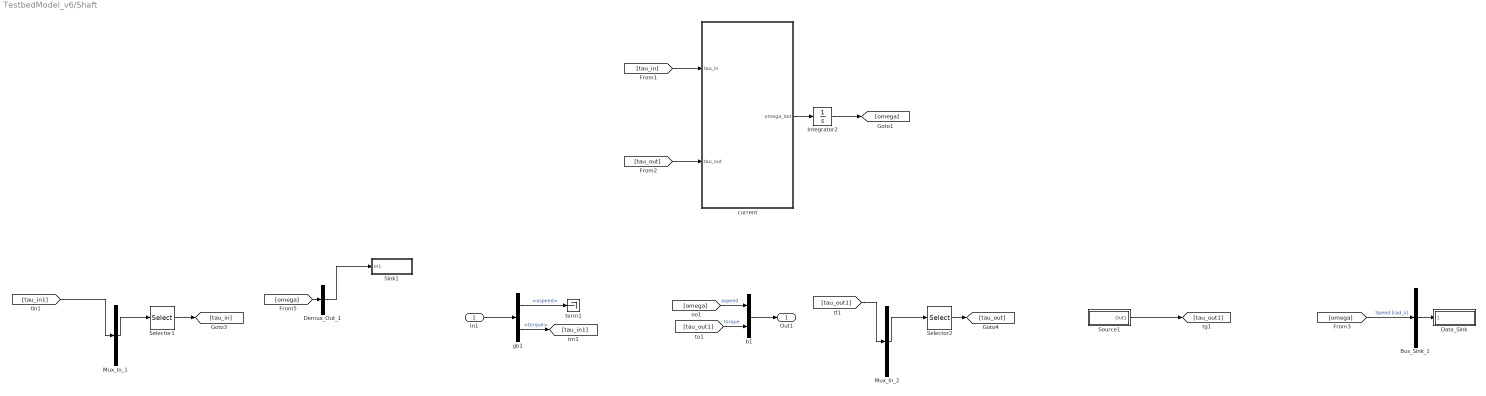
== system TestbedModel_v6/Shaft ==
  In1 : Inport
  Bus_Sink_1 : BusCreator  Inputs=1
  Data_Sink : Subsystem  LoadFcn=|  InitFcn=|  mask(Data Sink){}
      LoadFcn=|
      | h      = get_param(gcb,'handle');   % Get block handle                           
      | hblock = get(h);     % Parse out handles structure
      | 
      | str = [hblock.Path(numel(bdroot)+2:end), hblock.Name];
      | str(~ismember(str,['A':'Z' 'a':'z' '0':'9' '_'])) = '';                     
      | set_param([gcb, '/global_data_goto'],'GotoTag',['gdata_',str]);
      |                                
      |                                                                                  
      | clear h hblock str
      InitFcn=|
      | h      = get_param(gcb,'handle');   % Get block handle                           
      | hblock = get(h);     % Parse out handles structure
      | 
      | str = [hblock.Path(numel(bdroot)+2:end), hblock.Name];
      | str(~ismember(str,['A':'Z' 'a':'z' '0':'9' '_'])) = '';                     
      | set_param([gcb, '/global_data_goto'],'GotoTag',['gdata_',str]);
      |                                
      |                                                                                  
      | clear h hblock str
      mask help:
      | Input to this block should be a bus signal with named signals.
      |
      | Bus signals sent to this block will be read by the Data Manager.
      | The Data Manager will handle the global routing of signals.
      |
      | This block should be placed under the mask of components.
      settings: CopyFcn=|
      | h      = get_param(gcb,'handle');   % Get block handle
      | hblock = get(h);     % Parse out handles structure
      | 
      | str = [hblock.Path(numel(bdroot)+2:end), hblock.Name];
      | str(~ismember(str,['A':'Z' 'a':'z' '0':'9' '_'])) = '';
      | set_param([gcb, '/global_data_goto'],'GotoTag',['gdata_',str]);
      | 
      | 
      | clear h hblock str
      settings: NameChangeFcn=|
      | h      = get_param(gcb,'handle');   % Get block handle
      | hblock = get(h);     % Parse out handles structure
      | 
      | str = [hblock.Path(numel(bdroot)+2:end), hblock.Name];
      | str(~ismember(str,['A':'Z' 'a':'z' '0':'9' '_'])) = '';
      | set_param([gcb, '/global_data_goto'],'GotoTag',['gdata_',str]);
      | 
      | 
      | clear h hblock str
      mask Display: text(0.25,0.5,'Data Sink')
  Demux_Out_1 : Demux  Outputs=1
  Integrator2 : Integrator  InitialCondition=w_initial
  Mux_In_1 : Mux  Inputs=1
  Mux_In_2 : Mux  Inputs=1
  Selector1 : Selector  InputPortWidth=1  IndexOptions=Index vector (dialog)  Indices=[1 ]  OutputSizes=1
  Selector2 : Selector  InputPortWidth=1  IndexOptions=Index vector (dialog)  Indices=[1 ]  OutputSizes=1
  Sink1 : Subsystem  LoadFcn=rev_comms_sink();  InitFcn=rev_comms_sink();  mask(Sink){}
      mask help: Used for sending data to the upstream component.
      settings: CopyFcn=rev_comms_sink();  NameChangeFcn=rev_comms_sink();
      mask Display: text(0.25,0.5,'Sink')
  Source1 : Subsystem  mask(Source){}
      mask help: Used for receiving data from the downstream component.
      mask init:
      | n_src = gcb;
      | n_src = str2num(n_src(end));
      | try
      |     rev_comms_source(n_src);
      | catch
      | 
      | end
      mask Display: text(0.25,0.5,'Source')
  b1 : BusCreator  Inputs=2
  current : MATLAB Function  TreatAsAtomicUnit=on
  gb1 : BusSelector  OutputSignals=aspeed,torque
  term1 : Terminator
  Out1 : Outport
  wires:
  [omega] -> Bus_Sink_1/1  "Speed [rad_s]"
  Selector2/1 -> [tau_out]
  Selector1/1 -> [tau_in]
  b1/1 -> Out1/1
  Source1/1(Out1) -> [tau_out1]
  [omega] -> b1/1  "aspeed"
  [tau_out1] -> b1/2  "torque"
  Mux_In_2/1 -> Selector2/1
  [tau_out1] -> Mux_In_2/1
  Bus_Sink_1/1 -> Data_Sink/1(" ")
  current/1(omega_dot) -> Integrator2/1
  Mux_In_1/1 -> Selector1/1
  Integrator2/1 -> [omega]
  In1/1 -> gb1/1
  gb1/1 -> term1/1  "<aspeed>"
  gb1/2 -> [tau_in1]  "<torque>"
  [tau_in1] -> Mux_In_1/1
  [tau_in] -> current/1(tau_in)
  [tau_out] -> current/2(tau_out)
  Demux_Out_1/1 -> Sink1/1(In1)
  [omega] -> Demux_Out_1/1

== system TestbedModel_v6/State Machine ==
  Battery : Inport
  Bus Currents : Inport  Port=2
  Clock1 : Clock
  Clock2 : Clock
  Clock4 : Clock
  Demux : Demux  Outputs=5
  Demux3 : Demux  Outputs=2
  Memory4 : Memory  X0=[0,1,0]
  Memory6 : Memory  X0=[0]
  Memory7 : Memory  X0=1
  Mux1 : Mux  Inputs=3
  Mux2 : Mux  Inputs=3
  Mux7 : Mux
  Mux8 : Mux
  Output : MATLABFcn  MATLABFcn=Output  OutputDimensions=2  Output1D=off
  Reshape2 : Reshape  OutputDimensionality=Column vector (2-D)
  Reshape3 : Reshape  OutputDimensionality=Column vector (2-D)
  Reshape4 : Reshape  OutputDimensionality=Column vector (2-D)
  Scope : Scope
  Selector : Selector  InputPortWidth=4  IndexOptions=Index vector (dialog)  Indices=[1]  OutputSizes=1
  Selector1 : Selector  InputPortWidth=4  IndexOptions=Index vector (dialog)  Indices=[2:4]  OutputSizes=1
  hysteresis : MATLABFcn  MATLABFcn=hysteresis  OutputDimensions=4  Output1D=off
  stateLogic : MATLABFcn  MATLABFcn=stateLogic  OutputDimensions=5  Output1D=off
  I_lim : Outport
  Switch : Outport  Port=2
  state : Outport  Port=3
  wires:
  Reshape2/1 -> stateLogic/1
  Clock2/1 -> Mux7/1
  Demux/2 -> Memory6/1  "sw"
  Memory7/1 -> Scope/1, Mux8/3
  Clock4/1 -> Mux8/1
  Mux8/1 -> Reshape3/1
  Reshape3/1 -> hysteresis/1
  hysteresis/1 -> Selector1/1, Selector/1
  Memory4/1 -> Mux8/4
  Demux/1 -> Memory7/1, Mux8/2  "state"
  stateLogic/1 -> Demux/1
  Clock1/1 -> Mux1/1
  Reshape4/1 -> Output/1
  Mux1/1 -> Reshape4/1
  Selector/1 -> state/1, Mux1/3  "stateH"
  Output/1 -> Demux3/1
  Selector1/1 -> Memory4/1
  Battery/1 -> Mux7/2
  Bus Currents/1 -> Mux7/3
  Demux3/1 -> I_lim/1  "I_lim"
  Demux3/2 -> Switch/1  "Switch"
  Memory6/1 -> Mux7/4
  Mux7/1 -> Reshape2/1
  Demux/3 -> Mux2/1
  Demux/4 -> Mux2/2
  Demux/5 -> Mux2/3
  Mux2/1 -> Mux1/2

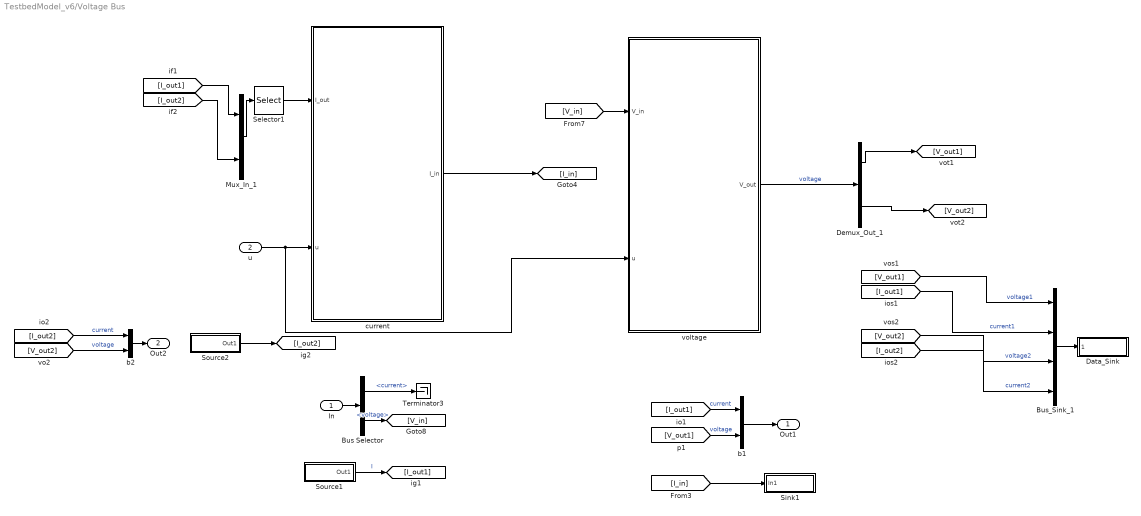
== system TestbedModel_v6/Voltage Bus ==
  In : Inport
  u : Inport  Port=2
  Bus Selector : BusSelector  OutputSignals=current,voltage
  Bus_Sink_1 : BusCreator  Inputs=4
  Data_Sink : Subsystem  LoadFcn=|  InitFcn=|  mask(Data Sink){}
      LoadFcn=|
      | h      = get_param(gcb,'handle');   % Get block handle                           
      | hblock = get(h);     % Parse out handles structure
      | 
      | str = [hblock.Path(numel(bdroot)+2:end), hblock.Name];
      | str(~ismember(str,['A':'Z' 'a':'z' '0':'9' '_'])) = '';                     
      | set_param([gcb, '/global_data_goto'],'GotoTag',['gdata_',str]);
      |                                
      |                                                                                  
      | clear h hblock str
      InitFcn=|
      | h      = get_param(gcb,'handle');   % Get block handle                           
      | hblock = get(h);     % Parse out handles structure
      | 
      | str = [hblock.Path(numel(bdroot)+2:end), hblock.Name];
      | str(~ismember(str,['A':'Z' 'a':'z' '0':'9' '_'])) = '';                     
      | set_param([gcb, '/global_data_goto'],'GotoTag',['gdata_',str]);
      |                                
      |                                                                                  
      | clear h hblock str
      mask help:
      | Input to this block should be a bus signal with named signals.
      |
      | Bus signals sent to this block will be read by the Data Manager.
      | The Data Manager will handle the global routing of signals.
      |
      | This block should be placed under the mask of components.
      settings: CopyFcn=|
      | h      = get_param(gcb,'handle');   % Get block handle
      | hblock = get(h);     % Parse out handles structure
      | 
      | str = [hblock.Path(numel(bdroot)+2:end), hblock.Name];
      | str(~ismember(str,['A':'Z' 'a':'z' '0':'9' '_'])) = '';
      | set_param([gcb, '/global_data_goto'],'GotoTag',['gdata_',str]);
      | 
      | 
      | clear h hblock str
      settings: NameChangeFcn=|
      | h      = get_param(gcb,'handle');   % Get block handle
      | hblock = get(h);     % Parse out handles structure
      | 
      | str = [hblock.Path(numel(bdroot)+2:end), hblock.Name];
      | str(~ismember(str,['A':'Z' 'a':'z' '0':'9' '_'])) = '';
      | set_param([gcb, '/global_data_goto'],'GotoTag',['gdata_',str]);
      | 
      | 
      | clear h hblock str
      mask Display: text(0.25,0.5,'Data Sink')
  Demux_Out_1 : Demux  Outputs=2
  Mux_In_1 : Mux  Inputs=2
  Selector1 : Selector  InputPortWidth=2  IndexOptions=Index vector (dialog)  Indices=[1 2 ]  OutputSizes=1
  Sink1 : Subsystem  LoadFcn=rev_comms_sink();  InitFcn=rev_comms_sink();  mask(Sink){}
      mask help: Used for sending data to the upstream component.
      settings: CopyFcn=rev_comms_sink();  NameChangeFcn=rev_comms_sink();
      mask Display: text(0.25,0.5,'Sink')
  Source1 : Subsystem  mask(Source){}
      mask help: Used for receiving data from the downstream component.
      mask init:
      | n_src = gcb;
      | n_src = str2num(n_src(end));
      | try
      |     rev_comms_source(n_src);
      | catch
      | 
      | end
      mask Display: text(0.25,0.5,'Source')
  Source2 : Subsystem  mask(Source){}
      mask help: Used for receiving data from the downstream component.
      mask init:
      | n_src = gcb;
      | n_src = str2num(n_src(end));
      | try
      |     rev_comms_source(n_src);
      | catch
      | 
      | end
      mask Display: text(0.25,0.5,'Source')
  Terminator3 : Terminator
  b1 : BusCreator  Inputs=2
  b2 : BusCreator  Inputs=2
  current : MATLAB Function  TreatAsAtomicUnit=on
  voltage : MATLAB Function  TreatAsAtomicUnit=on
  Out1 : Outport
  Out2 : Outport  Port=2
  wires:
  Demux_Out_1/2 -> [V_out2]
  [I_out2] -> Mux_In_1/2
  Source2/1(Out1) -> [I_out2]
  b2/1 -> Out2/1
  [I_out2] -> Bus_Sink_1/4  "current2"
  [V_out2] -> Bus_Sink_1/3  "voltage2"
  [V_out2] -> b2/2  "voltage"
  [I_out2] -> b2/1  "current"
  [I_out1] -> Bus_Sink_1/2  "current1"
  [V_out1] -> Bus_Sink_1/1  "voltage1"
  Demux_Out_1/1 -> [V_out1]
  [V_in] -> voltage/1(V_in)
  Selector1/1 -> current/1(I_out)
  u/1 -> voltage/2(u), current/2(u)
  Bus_Sink_1/1 -> Data_Sink/1(" ")
  current/1(I_in) -> [I_in]
  [I_out1] -> Mux_In_1/1
  Mux_In_1/1 -> Selector1/1
  voltage/1(V_out) -> Demux_Out_1/1  "voltage"
  [V_out1] -> b1/2  "voltage"
  [I_out1] -> b1/1  "current"
  [I_in] -> Sink1/1(In1)
  Source1/1(Out1) -> [I_out1]  "I"
  Bus Selector/2 -> [V_in]  "<voltage>"
  Bus Selector/1 -> Terminator3/1  "<current>"
  In/1 -> Bus Selector/1
  b1/1 -> Out1/1

== system TestbedModel_v6/Air Vehicle/Data_Sink ==
  " " : Inport
  tag scope: gdata_AirVehicleData_Sink=global
  wires:
  " "/1 -> [gdata_AirVehicleData_Sink]

== system TestbedModel_v6/Air Vehicle/Property ==
  v : Inport
  w : Inport  Port=2
  2-D Lookup Table : Lookup_n-D  BreakpointsForDimension1=Prop.omega  BreakpointsForDimension2=Prop.v  Table=Prop.CT_2D  InternalRulePriority=Speed  RndMeth=Simplest  InputSameDT=on
  Divide : Product  Inputs=/*
  Gain : Gain  Gain=d
  Gain1 : Gain  Gain=2*pi
  Scope : Scope
  Scope1 : Scope
  Props : Outport
  wires:
  2-D Lookup Table/1 -> Scope/1, Props/1  "C_T"
  w/1 -> Gain/1, 2-D Lookup Table/1
  v/1 -> Gain1/1, 2-D Lookup Table/2
  Gain/1 -> Divide/1
  Gain1/1 -> Divide/2
  Divide/1 -> Scope1/1

== system TestbedModel_v6/Air Vehicle/Sink1 ==
  In1 : Inport
  tag scope: gdata_TestbedModel_v6AirVehicleSink1=global
  wires:
  In1/1 -> [gdata_TestbedModel_v6AirVehicleSink1]

== system TestbedModel_v6/Battery/Data_Sink ==
  " " : Inport
  tag scope: gdata_BatteryData_Sink=global
  wires:
  " "/1 -> [gdata_BatteryData_Sink]

== system TestbedModel_v6/Battery/Property ==
  I : Inport
  T_m : Inport  Port=2
  SOC : Inport  Port=3
  " " : Lookup  InputValues=cell.Ent_SOC  Table=cell.dUdt
  " " : Lookup  InputValues=cell.V_SOC  Table=cell.Vocv  LookUpMeth=Interpolation-Use End Values
  Fcn{1..5} (5 alike) : Fcn  Expr=((u(1)-u(3))/(1+exp(-50*u(2))))+u(3)
  Gain : Gain  Gain=Ns
  Mux : Mux  Inputs=7
  Mux{1..5} (5 alike) : Mux  Inputs=3
  n-D Lookup Table1 : Lookup_n-D  BreakpointsForDimension1=cell.RC_SOC_c  BreakpointsForDimension2=cell.Temp  BreakpointsForDimension3=[5, 7]  Table=cell.Rs_c  RndMeth=Simplest  InputSameDT=on
  n-D Lookup Table13 : Lookup_n-D  BreakpointsForDimension1=cell.RC_SOC_d  BreakpointsForDimension2=cell.Temp  BreakpointsForDimension3=[5, 7]  Table=cell.Rs_d  RndMeth=Simplest  InputSameDT=on
  n-D Lookup Table2 : Lookup_n-D  BreakpointsForDimension1=cell.RC_SOC_d  BreakpointsForDimension2=cell.Temp  BreakpointsForDimension3=[5, 7]  Table=cell.R1_d  RndMeth=Simplest  InputSameDT=on
  n-D Lookup Table3 : Lookup_n-D  BreakpointsForDimension1=cell.RC_SOC_c  BreakpointsForDimension2=cell.Temp  BreakpointsForDimension3=[5, 7]  Table=cell.R1_c  RndMeth=Simplest  InputSameDT=on
  n-D Lookup Table4 : Lookup_n-D  BreakpointsForDimension1=cell.RC_SOC_d  BreakpointsForDimension2=cell.Temp  BreakpointsForDimension3=[5, 7]  Table=cell.C1_d  RndMeth=Simplest  InputSameDT=on
  n-D Lookup Table5 : Lookup_n-D  BreakpointsForDimension1=cell.RC_SOC_c  BreakpointsForDimension2=cell.Temp  BreakpointsForDimension3=[5, 7]  Table=cell.C1_c  RndMeth=Simplest  InputSameDT=on
  n-D Lookup Table6 : Lookup_n-D  BreakpointsForDimension1=cell.RC_SOC_d  BreakpointsForDimension2=cell.Temp  BreakpointsForDimension3=[5, 7]  Table=cell.R2_d  RndMeth=Simplest  InputSameDT=on
  n-D Lookup Table7 : Lookup_n-D  BreakpointsForDimension1=cell.RC_SOC_c  BreakpointsForDimension2=cell.Temp  BreakpointsForDimension3=[5, 7]  Table=cell.R2_c  RndMeth=Simplest  InputSameDT=on
  n-D Lookup Table8 : Lookup_n-D  BreakpointsForDimension1=cell.RC_SOC_d  BreakpointsForDimension2=cell.Temp  BreakpointsForDimension3=[5, 7]  Table=cell.C2_d  RndMeth=Simplest  InputSameDT=on
  n-D Lookup Table9 : Lookup_n-D  BreakpointsForDimension1=cell.RC_SOC_c  BreakpointsForDimension2=cell.Temp  BreakpointsForDimension3=[5, 7]  Table=cell.C2_c  RndMeth=Simplest  InputSameDT=on
  Props : Outport
  wires:
  n-D Lookup Table9/1 -> Mux5/3
  n-D Lookup Table8/1 -> Mux5/1
  Mux5/1 -> Fcn5/1
  n-D Lookup Table7/1 -> Mux4/3
  n-D Lookup Table6/1 -> Mux4/1
  Mux4/1 -> Fcn4/1
  n-D Lookup Table5/1 -> Mux3/3
  n-D Lookup Table4/1 -> Mux3/1
  Mux3/1 -> Fcn3/1
  n-D Lookup Table3/1 -> Mux1/3
  n-D Lookup Table2/1 -> Mux1/1
  Mux1/1 -> Fcn2/1
  n-D Lookup Table13/1 -> Mux2/1
  n-D Lookup Table1/1 -> Mux2/3
  Mux2/1 -> Fcn1/1
  Fcn3/1 -> Mux/3  "C1"
  Fcn2/1 -> Mux/2  "R1"
  Fcn4/1 -> Mux/4  "R2"
  Fcn5/1 -> Mux/5  "C2"
  I/1 -> Mux3/2, Mux4/2, Mux5/2, Mux1/2, Mux2/2
  SOC/1 -> n-D Lookup Table13/1, n-D Lookup Table1/1, n-D Lookup Table2/1, n-D Lookup Table3/1, n-D Lookup Table4/1, n-D Lookup Table5/1, n-D Lookup Table6/1, n-D Lookup Table7/1, n-D Lookup Table8/1, " "/1, " "/1, n-D Lookup Table9/1
  T_m/1 -> n-D Lookup Table13/2, n-D Lookup Table1/2, n-D Lookup Table2/2, n-D Lookup Table3/2, n-D Lookup Table4/2, n-D Lookup Table5/2, n-D Lookup Table6/2, n-D Lookup Table7/2, n-D Lookup Table8/2, n-D Lookup Table9/2
  Fcn1/1 -> Mux/1  "Rs"
  " "/1 -> Mux/6  "dU_dt"
  " "/1 -> Gain/1  "V_ocv"
  Mux/1 -> Props/1
  Gain/1 -> Mux/7

== system TestbedModel_v6/Battery/Sink1 ==
  In1 : Inport
  tag scope: gdata_TestbedModel_v6BatterySink1=global
  wires:
  In1/1 -> [gdata_TestbedModel_v6BatterySink1]

== system TestbedModel_v6/Battery/Source1 ==
  Out1 : Outport
  wires:
  [gdata_TestbedModel_v6BusSink1] -> Out1/1

== system TestbedModel_v6/Battery/Source2 ==
  Out1 : Outport
  wires:
  [gdata_TestbedModel_v6EffortSink14Sink1] -> Out1/1

== system TestbedModel_v6/Bus/Data_Sink ==
  " " : Inport
  tag scope: gdata_BusData_Sink=global
  wires:
  " "/1 -> [gdata_BusData_Sink]
